simulink model "main"  (R2021a)
settings: Solver=ode113  StartTime=0.0  StopTime=300  RelTol=1e-13  AbsTol=1e-14
values from neighbouring files (symbols this model uses):
  Const = createSimulinkBus(Const_1)    [initializeData.m]
  Earth = createSimulinkBus(Earth_1)    [initializeData.m]
  Sensors = createSimulinkBus(Sensors_1)    [initializeData.m]
  Spacecraft = createSimulinkBus(Spacecraft_1)    [initializeData.m]
  totalTorque = [0 0 0 0.000704944678681 0.000834848489248 0.000628617928475 0.000704944678681 -0.000834848489248 -0.000628617928475 0.00140988935736 0 0 ... (48 elements, 3x16)]    [totalTorque.mat]
undefined symbols (not defined in the file or in its folder): initCond, torqueLookUpTable
libraries: simulink x22, SADlibrary x22, aerolibutil x20, vrlib x14, dspsrcs4 x12, sharedtransform x5, commfilt2 x3, dspfdesign x3, simulink_extras x2, sharedTrackingLibrary x2, dspmathops x1, sharedutil x1
(part 2 of 2)

== system main/Star sensor/Vector 2 angles ==
  In1 : Inport
  Atan1 : Trigonometry  Operator=atan2
  Atan2 : Trigonometry  Operator=atan2
  Demux : Demux  Outputs=3
  Mux : Mux  Inputs=2
  Random Source : dspsrcs4/Random Source  SrcType=Gaussian  NormMethod=Ziggurat  CltLength=12  MinVal=0  MaxVal=1  MeanVal=0  VarVal=Sensors.starTrackerCovariance  RepMode=Not repeatable  rawSeed=1  IsInherit=off  SampMode=Discrete  SampTime=1/Sensors.starTrackerSamplingFreq  SampFrame=2  DataType=Double  OutComplex=Real  OutputFrames=off
  Sum : Sum  Inputs=|++
  Star 1 : Outport
  wires:
  In1/1 -> Demux/1
  Sum/1 -> Star 1/1
  Mux/1 -> Sum/1
  Atan1/1 -> Mux/2
  Random Source/1 -> Sum/2
  Demux/3 -> Atan2/2, Atan1/2
  Atan2/1 -> Mux/1
  Demux/2 -> Atan1/1
  Demux/1 -> Atan2/1

== system main/Star sensor/Vector 2 angles1 ==
  In1 : Inport
  Atan1 : Trigonometry  Operator=atan2
  Atan2 : Trigonometry  Operator=atan2
  Demux : Demux  Outputs=3
  Mux : Mux  Inputs=2
  Random Source : dspsrcs4/Random Source  SrcType=Gaussian  NormMethod=Ziggurat  CltLength=12  MinVal=0  MaxVal=1  MeanVal=0  VarVal=Sensors.starTrackerCovariance  RepMode=Not repeatable  rawSeed=1  IsInherit=off  SampMode=Discrete  SampTime=1/Sensors.starTrackerSamplingFreq  SampFrame=2  DataType=Double  OutComplex=Real  OutputFrames=off
  Sum : Sum  Inputs=|++
  Star 1 : Outport
  wires:
  In1/1 -> Demux/1
  Sum/1 -> Star 1/1
  Mux/1 -> Sum/1
  Atan1/1 -> Mux/2
  Random Source/1 -> Sum/2
  Demux/3 -> Atan2/2, Atan1/2
  Atan2/1 -> Mux/1
  Demux/2 -> Atan1/1
  Demux/1 -> Atan2/1

== system main/Star sensor/Vector 2 angles2 ==
  In1 : Inport
  Atan1 : Trigonometry  Operator=atan2
  Atan2 : Trigonometry  Operator=atan2
  Demux : Demux  Outputs=3
  Mux : Mux  Inputs=2
  Random Source : dspsrcs4/Random Source  SrcType=Gaussian  NormMethod=Ziggurat  CltLength=12  MinVal=0  MaxVal=1  MeanVal=0  VarVal=Sensors.starTrackerCovariance  RepMode=Not repeatable  rawSeed=1  IsInherit=off  SampMode=Discrete  SampTime=1/Sensors.starTrackerSamplingFreq  SampFrame=2  DataType=Double  OutComplex=Real  OutputFrames=off
  Sum : Sum  Inputs=|++
  Star 1 : Outport
  wires:
  In1/1 -> Demux/1
  Sum/1 -> Star 1/1
  Mux/1 -> Sum/1
  Atan1/1 -> Mux/2
  Random Source/1 -> Sum/2
  Demux/3 -> Atan2/2, Atan1/2
  Atan2/1 -> Mux/1
  Demux/2 -> Atan1/1
  Demux/1 -> Atan2/1

== system main/Star sensor/Vector 2 angles3 ==
  In1 : Inport
  Atan1 : Trigonometry  Operator=atan2
  Atan2 : Trigonometry  Operator=atan2
  Demux : Demux  Outputs=3
  Mux : Mux  Inputs=2
  Random Source : dspsrcs4/Random Source  SrcType=Gaussian  NormMethod=Ziggurat  CltLength=12  MinVal=0  MaxVal=1  MeanVal=0  VarVal=Sensors.starTrackerCovariance  RepMode=Not repeatable  rawSeed=1  IsInherit=off  SampMode=Discrete  SampTime=1/Sensors.starTrackerSamplingFreq  SampFrame=2  DataType=Double  OutComplex=Real  OutputFrames=off
  Sum : Sum  Inputs=|++
  Star 1 : Outport
  wires:
  In1/1 -> Demux/1
  Sum/1 -> Star 1/1
  Mux/1 -> Sum/1
  Atan1/1 -> Mux/2
  Random Source/1 -> Sum/2
  Demux/3 -> Atan2/2, Atan1/2
  Atan2/1 -> Mux/1
  Demux/2 -> Atan1/1
  Demux/1 -> Atan2/1

== system main/State estimator/State 2 attitude and bias ==
  xHat : Inport
  Demux1 : Demux  Outputs=7
  Mux2 : Mux
  Mux3 : Mux  Inputs=3
  Body frame attitude [ECI] : Outport
  Gyro bias [body frame] : Outport  Port=2
  wires:
  Mux2/1 -> Body frame attitude [ECI]/1
  Demux1/2 -> Mux2/2
  Mux3/1 -> Gyro bias [body frame]/1
  Demux1/7 -> Mux3/3
  Demux1/1 -> Mux2/1
  Demux1/3 -> Mux2/3
  Demux1/5 -> Mux3/1
  xHat/1 -> Demux1/1
  Demux1/6 -> Mux3/2
  Demux1/4 -> Mux2/4

== system main/State estimator/State 2 attitude and bias1 ==
  xHat : Inport
  Demux1 : Demux  Outputs=7
  Mux2 : Mux
  Mux3 : Mux  Inputs=3
  Body frame attitude [ECI] : Outport
  Gyro bias [body frame] : Outport  Port=2
  wires:
  Mux2/1 -> Body frame attitude [ECI]/1
  Demux1/2 -> Mux2/2
  Mux3/1 -> Gyro bias [body frame]/1
  Demux1/7 -> Mux3/3
  Demux1/1 -> Mux2/1
  Demux1/3 -> Mux2/3
  Demux1/5 -> Mux3/1
  xHat/1 -> Demux1/1
  Demux1/6 -> Mux3/2
  Demux1/4 -> Mux2/4

== system main/Subsystem/Vec norm ==
  Vector : Inport
  Sqrt1 : Sqrt  SaturateOnIntegerOverflow=on
  Square : Math  Operator=square  SaturateOnIntegerOverflow=on
  Sum of Elements : Sum  Inputs=+
  Length : Outport
  wires:
  Sqrt1/1 -> Length/1
  Sum of Elements/1 -> Sqrt1/1
  Vector/1 -> Square/1
  Square/1 -> Sum of Elements/1

== system main/Subsystem/Vec norm1 ==
  Vector : Inport
  Sqrt1 : Sqrt  SaturateOnIntegerOverflow=on
  Square : Math  Operator=square  SaturateOnIntegerOverflow=on
  Sum of Elements : Sum  Inputs=+
  Length : Outport
  wires:
  Sqrt1/1 -> Length/1
  Sum of Elements/1 -> Sqrt1/1
  Vector/1 -> Square/1
  Square/1 -> Sum of Elements/1

== system main/Subsystem/Vec norm2 ==
  Vector : Inport
  Sqrt1 : Sqrt  SaturateOnIntegerOverflow=on
  Square : Math  Operator=square  SaturateOnIntegerOverflow=on
  Sum of Elements : Sum  Inputs=+
  Length : Outport
  wires:
  Sqrt1/1 -> Length/1
  Sum of Elements/1 -> Sqrt1/1
  Vector/1 -> Square/1
  Square/1 -> Sum of Elements/1

== system main/Subsystem1/Sun sensor reading1 ==
  True Sun position [body reference frame][km] : Inport  OutDataTypeStr=double  Unit=km
  Atan1 : Trigonometry  Operator=atan2
  Atan2 : Trigonometry  Operator=atan2
  Constant : Constant  Value=0*.5*pi/180*randn(2,1)
  Demux1 : Demux  Outputs=3
  Mux : Mux  Inputs=2
  Normalize Vector : vrlib/Utilities/Normalize Vector  maxzero=0
  Quaternion Rotation : aerolibutil/Quaternion Rotation
  Random Source1 : dspsrcs4/Random Source  SrcType=Gaussian  NormMethod=Ziggurat  CltLength=12  MinVal=0  MaxVal=1  MeanVal=0  VarVal=(.1*pi/180)^2  RepMode=Not repeatable  rawSeed=1  IsInherit=off  SampMode=Discrete  SampTime=Sensors.sunSensorSamplingFreq  SampFrame=2  DataType=Double  OutComplex=Real  OutputFrames=off
  Saturation : Saturate  UpperLimit=60*pi/180  LowerLimit=-60*pi/180
  Sensor orientation : Constant  Value=[1 0 0 0]
  Sum : Sum  Inputs=|++
  Sum1 : Sum  Inputs=++|
  Zero-Order Hold : ZeroOrderHold  SampleTime=Sensors.sunSensorSamplingFreq
  Sun angles position [sensor axis] : Outport  OutDataTypeStr=double  Unit=1
  wires:
  True Sun position [body reference frame][km]/1 -> Zero-Order Hold/1
  Sensor orientation/1 -> Quaternion Rotation/1
  Zero-Order Hold/1 -> Normalize Vector/1
  Normalize Vector/1 -> Quaternion Rotation/2
  Quaternion Rotation/1 -> Demux1/1
  Demux1/1 -> Atan2/1
  Demux1/3 -> Atan1/2, Atan2/2
  Demux1/2 -> Atan1/1
  Atan2/1 -> Mux/1
  Atan1/1 -> Mux/2
  Constant/1 -> Sum1/1
  Mux/1 -> Sum1/2
  Saturation/1 -> Sun angles position [sensor axis]/1
  Random Source1/1 -> Sum/2
  Sum/1 -> Saturation/1
  Sum1/1 -> Sum/1

== system main/Subsystem1/Sun sensor reading2 ==
  True Sun position [body reference frame][km] : Inport  OutDataTypeStr=double  Unit=km
  Atan1 : Trigonometry  Operator=atan2
  Atan2 : Trigonometry  Operator=atan2
  Constant : Constant  Value=0*.5*pi/180*randn(2,1)
  Demux1 : Demux  Outputs=3
  Mux : Mux  Inputs=2
  Normalize Vector : vrlib/Utilities/Normalize Vector  maxzero=0
  Quaternion Rotation : aerolibutil/Quaternion Rotation
  Random Source1 : dspsrcs4/Random Source  SrcType=Gaussian  NormMethod=Ziggurat  CltLength=12  MinVal=0  MaxVal=1  MeanVal=0  VarVal=(.1*pi/180)^2  RepMode=Not repeatable  rawSeed=1  IsInherit=off  SampMode=Discrete  SampTime=Sensors.sunSensorSamplingFreq  SampFrame=2  DataType=Double  OutComplex=Real  OutputFrames=off
  Saturation : Saturate  UpperLimit=60*pi/180  LowerLimit=-60*pi/180
  Sensor orientation : Constant  Value=[cos(pi/4) sin(pi/4) 0 0]
  Sum : Sum  Inputs=|++
  Sum1 : Sum  Inputs=++|
  Zero-Order Hold : ZeroOrderHold  SampleTime=Sensors.sunSensorSamplingFreq
  Sun angles position [sensor axis] : Outport  OutDataTypeStr=double  Unit=1
  wires:
  True Sun position [body reference frame][km]/1 -> Zero-Order Hold/1
  Sensor orientation/1 -> Quaternion Rotation/1
  Zero-Order Hold/1 -> Normalize Vector/1
  Normalize Vector/1 -> Quaternion Rotation/2
  Quaternion Rotation/1 -> Demux1/1
  Demux1/1 -> Atan2/1
  Demux1/3 -> Atan1/2, Atan2/2
  Demux1/2 -> Atan1/1
  Atan2/1 -> Mux/1
  Atan1/1 -> Mux/2
  Constant/1 -> Sum1/1
  Mux/1 -> Sum1/2
  Saturation/1 -> Sun angles position [sensor axis]/1
  Random Source1/1 -> Sum/2
  Sum/1 -> Saturation/1
  Sum1/1 -> Sum/1

== system main/Subsystem1/Sun sensor reading3 ==
  True Sun position [body reference frame][km] : Inport  OutDataTypeStr=double  Unit=km
  Atan1 : Trigonometry  Operator=atan2
  Atan2 : Trigonometry  Operator=atan2
  Constant : Constant  Value=0*.5*pi/180*randn(2,1)
  Demux1 : Demux  Outputs=3
  Mux : Mux  Inputs=2
  Normalize Vector : vrlib/Utilities/Normalize Vector  maxzero=0
  Quaternion Rotation : aerolibutil/Quaternion Rotation
  Random Source1 : dspsrcs4/Random Source  SrcType=Gaussian  NormMethod=Ziggurat  CltLength=12  MinVal=0  MaxVal=1  MeanVal=0  VarVal=(.1*pi/180)^2  RepMode=Not repeatable  rawSeed=1  IsInherit=off  SampMode=Discrete  SampTime=Sensors.sunSensorSamplingFreq  SampFrame=2  DataType=Double  OutComplex=Real  OutputFrames=off
  Saturation : Saturate  UpperLimit=60*pi/180  LowerLimit=-60*pi/180
  Sensor orientation : Constant  Value=[cos(pi/2) sin(pi/2) 0 0]
  Sum : Sum  Inputs=|++
  Sum1 : Sum  Inputs=++|
  Zero-Order Hold : ZeroOrderHold  SampleTime=Sensors.sunSensorSamplingFreq
  Sun angles position [sensor axis] : Outport  OutDataTypeStr=double  Unit=1
  wires:
  True Sun position [body reference frame][km]/1 -> Zero-Order Hold/1
  Sensor orientation/1 -> Quaternion Rotation/1
  Zero-Order Hold/1 -> Normalize Vector/1
  Normalize Vector/1 -> Quaternion Rotation/2
  Quaternion Rotation/1 -> Demux1/1
  Demux1/1 -> Atan2/1
  Demux1/3 -> Atan1/2, Atan2/2
  Demux1/2 -> Atan1/1
  Atan2/1 -> Mux/1
  Atan1/1 -> Mux/2
  Constant/1 -> Sum1/1
  Mux/1 -> Sum1/2
  Saturation/1 -> Sun angles position [sensor axis]/1
  Random Source1/1 -> Sum/2
  Sum/1 -> Saturation/1
  Sum1/1 -> Sum/1

== system main/Subsystem1/Sun sensor reading4 ==
  True Sun position [body reference frame][km] : Inport  OutDataTypeStr=double  Unit=km
  Atan1 : Trigonometry  Operator=atan2
  Atan2 : Trigonometry  Operator=atan2
  Constant : Constant  Value=0*.5*pi/180*randn(2,1)
  Demux1 : Demux  Outputs=3
  Mux : Mux  Inputs=2
  Normalize Vector : vrlib/Utilities/Normalize Vector  maxzero=0
  Quaternion Rotation : aerolibutil/Quaternion Rotation
  Random Source1 : dspsrcs4/Random Source  SrcType=Gaussian  NormMethod=Ziggurat  CltLength=12  MinVal=0  MaxVal=1  MeanVal=0  VarVal=(.1*pi/180)^2  RepMode=Not repeatable  rawSeed=1  IsInherit=off  SampMode=Discrete  SampTime=Sensors.sunSensorSamplingFreq  SampFrame=2  DataType=Double  OutComplex=Real  OutputFrames=off
  Saturation : Saturate  UpperLimit=60*pi/180  LowerLimit=-60*pi/180
  Sensor orientation : Constant  Value=[cos(pi/4) -sin(pi/4) 0 0]
  Sum : Sum  Inputs=|++
  Sum1 : Sum  Inputs=++|
  Zero-Order Hold : ZeroOrderHold  SampleTime=Sensors.sunSensorSamplingFreq
  Sun angles position [sensor axis] : Outport  OutDataTypeStr=double  Unit=1
  wires:
  True Sun position [body reference frame][km]/1 -> Zero-Order Hold/1
  Sensor orientation/1 -> Quaternion Rotation/1
  Zero-Order Hold/1 -> Normalize Vector/1
  Normalize Vector/1 -> Quaternion Rotation/2
  Quaternion Rotation/1 -> Demux1/1
  Demux1/1 -> Atan2/1
  Demux1/3 -> Atan1/2, Atan2/2
  Demux1/2 -> Atan1/1
  Atan2/1 -> Mux/1
  Atan1/1 -> Mux/2
  Constant/1 -> Sum1/1
  Mux/1 -> Sum1/2
  Saturation/1 -> Sun angles position [sensor axis]/1
  Random Source1/1 -> Sum/2
  Sum/1 -> Saturation/1
  Sum1/1 -> Sum/1

== system main/Subsystem1/Sun sensor reading5 ==
  True Sun position [body reference frame][km] : Inport  OutDataTypeStr=double  Unit=km
  Atan1 : Trigonometry  Operator=atan2
  Atan2 : Trigonometry  Operator=atan2
  Constant : Constant  Value=0*.5*pi/180*randn(2,1)
  Demux1 : Demux  Outputs=3
  Mux : Mux  Inputs=2
  Normalize Vector : vrlib/Utilities/Normalize Vector  maxzero=0
  Quaternion Rotation : aerolibutil/Quaternion Rotation
  Random Source1 : dspsrcs4/Random Source  SrcType=Gaussian  NormMethod=Ziggurat  CltLength=12  MinVal=0  MaxVal=1  MeanVal=0  VarVal=(.1*pi/180)^2  RepMode=Not repeatable  rawSeed=1  IsInherit=off  SampMode=Discrete  SampTime=Sensors.sunSensorSamplingFreq  SampFrame=2  DataType=Double  OutComplex=Real  OutputFrames=off
  Saturation : Saturate  UpperLimit=60*pi/180  LowerLimit=-60*pi/180
  Sensor orientation : Constant  Value=[cos(pi/4) 0 sin(pi/4) 0]
  Sum : Sum  Inputs=|++
  Sum1 : Sum  Inputs=++|
  Zero-Order Hold : ZeroOrderHold  SampleTime=Sensors.sunSensorSamplingFreq
  Sun angles position [sensor axis] : Outport  OutDataTypeStr=double  Unit=1
  wires:
  True Sun position [body reference frame][km]/1 -> Zero-Order Hold/1
  Sensor orientation/1 -> Quaternion Rotation/1
  Zero-Order Hold/1 -> Normalize Vector/1
  Normalize Vector/1 -> Quaternion Rotation/2
  Quaternion Rotation/1 -> Demux1/1
  Demux1/1 -> Atan2/1
  Demux1/3 -> Atan1/2, Atan2/2
  Demux1/2 -> Atan1/1
  Atan2/1 -> Mux/1
  Atan1/1 -> Mux/2
  Constant/1 -> Sum1/1
  Mux/1 -> Sum1/2
  Saturation/1 -> Sun angles position [sensor axis]/1
  Random Source1/1 -> Sum/2
  Sum/1 -> Saturation/1
  Sum1/1 -> Sum/1

== system main/Subsystem1/Sun sensor reading6 ==
  True Sun position [body reference frame][km] : Inport  OutDataTypeStr=double  Unit=km
  Atan1 : Trigonometry  Operator=atan2
  Atan2 : Trigonometry  Operator=atan2
  Constant : Constant  Value=0*.5*pi/180*randn(2,1)
  Demux1 : Demux  Outputs=3
  Mux : Mux  Inputs=2
  Normalize Vector : vrlib/Utilities/Normalize Vector  maxzero=0
  Quaternion Rotation : aerolibutil/Quaternion Rotation
  Random Source1 : dspsrcs4/Random Source  SrcType=Gaussian  NormMethod=Ziggurat  CltLength=12  MinVal=0  MaxVal=1  MeanVal=0  VarVal=(.1*pi/180)^2  RepMode=Not repeatable  rawSeed=1  IsInherit=off  SampMode=Discrete  SampTime=Sensors.sunSensorSamplingFreq  SampFrame=2  DataType=Double  OutComplex=Real  OutputFrames=off
  Saturation : Saturate  UpperLimit=60*pi/180  LowerLimit=-60*pi/180
  Sensor orientation : Constant  Value=[cos(pi/4) 0 -sin(pi/4) 0]
  Sum : Sum  Inputs=|++
  Sum1 : Sum  Inputs=++|
  Zero-Order Hold : ZeroOrderHold  SampleTime=Sensors.sunSensorSamplingFreq
  Sun angles position [sensor axis] : Outport  OutDataTypeStr=double  Unit=1
  wires:
  True Sun position [body reference frame][km]/1 -> Zero-Order Hold/1
  Sensor orientation/1 -> Quaternion Rotation/1
  Zero-Order Hold/1 -> Normalize Vector/1
  Normalize Vector/1 -> Quaternion Rotation/2
  Quaternion Rotation/1 -> Demux1/1
  Demux1/1 -> Atan2/1
  Demux1/3 -> Atan1/2, Atan2/2
  Demux1/2 -> Atan1/1
  Atan2/1 -> Mux/1
  Atan1/1 -> Mux/2
  Constant/1 -> Sum1/1
  Mux/1 -> Sum1/2
  Saturation/1 -> Sun angles position [sensor axis]/1
  Random Source1/1 -> Sum/2
  Sum/1 -> Saturation/1
  Sum1/1 -> Sum/1

== system main/Real physics/Air drag/Air density ==
  note: Because the density is a continuous function it doesn't matter if with an Height equal to a breakpoint value (e.g. =700km) we consider a base height of 700km or a base height of 600km
  Height : Inport
  1-D Lookup Base height : Lookup_n-D  NumberOfTableDimensions=1  BreakpointsForDimension1=Earth.atm_referenceHeight  IndexSearchMethod=Evenly spaced points  BeginIndexSearchUsingPreviousIndexResult=on  Table=Earth.atm_referenceHeight  InterpMethod=Flat  ExtrapMethod=Clip  UseLastTableValue=on  InternalRulePriority=Speed  RndMeth=Simplest  InputSameDT=on
  1-D Lookup Nominal density : Lookup_n-D  NumberOfTableDimensions=1  BreakpointsForDimension1=Earth.atm_referenceHeight  IndexSearchMethod=Evenly spaced points  BeginIndexSearchUsingPreviousIndexResult=on  Table=Earth.atm_nominalDensity  InterpMethod=Flat  InternalRulePriority=Speed  RndMeth=Simplest  InputSameDT=on
  1-D Lookup Scale height : Lookup_n-D  NumberOfTableDimensions=1  BreakpointsForDimension1=Earth.atm_referenceHeight  IndexSearchMethod=Evenly spaced points  BeginIndexSearchUsingPreviousIndexResult=on  Table=Earth.atm_scaleHeight  InterpMethod=Flat  InternalRulePriority=Speed  RndMeth=Simplest  InputSameDT=on
  Divide : Product  Inputs=*/
  Exp : Math  SaturateOnIntegerOverflow=on
  Product : Product
  Sum : Sum  Inputs=-+|
  Air density : Outport
  wires:
  Height/1 -> 1-D Lookup Nominal density/1, 1-D Lookup Scale height/1, 1-D Lookup Base height/1, Sum/1
  1-D Lookup Nominal density/1 -> Product/2
  1-D Lookup Base height/1 -> Sum/2
  Sum/1 -> Divide/1
  1-D Lookup Scale height/1 -> Divide/2
  Divide/1 -> Exp/1
  Product/1 -> Air density/1
  Exp/1 -> Product/1

== system main/Real physics/Magnetic effect (torque only)/Cartesian to polar ==
  Unitary vector [cartesian coord] : Inport
  Atan1 : Trigonometry  Operator=atan2
  Atan2 : Trigonometry  Operator=atan2
  Demux : Demux  Outputs=3
  Sqrt : Sqrt  SaturateOnIntegerOverflow=on
  Square : Math  Operator=square  SaturateOnIntegerOverflow=on
  Square1 : Math  Operator=square  SaturateOnIntegerOverflow=on
  Sum : Sum
  Colatitude - θ : Outport
  Longitude - φ : Outport  Port=2
  wires:
  Demux/2 -> Square1/1, Atan2/1
  Square/1 -> Sum/1
  Square1/1 -> Sum/2
  Atan1/1 -> Colatitude - θ/1
  Sum/1 -> Sqrt/1
  Unitary vector [cartesian coord]/1 -> Demux/1
  Demux/1 -> Square/1, Atan2/2
  Demux/3 -> Atan1/2
  Atan2/1 -> Longitude - φ/1
  Sqrt/1 -> Atan1/1

== system main/Real physics/Rotational dynamic/Euler equations (rigid body)  ==
  note: $\dot\mathbf{\Gamma} = \left[ (-I_z+I_y) \omega_y \omega_z \quad (-I_x+I_z) \omega_z \omega_x \quad \right (-I_y+I_x) \omega_x \omega_y]^T$
      |
      | Please note that
      | $\left[b \quad c \quad a \right] = \text{Cycle_3_vector}\left([a \quad b \quad c]\right)$
  omega [body reference frame] : Inport
  Inertia [body reference frame] : Inport  Port=2  Unit=kg*m^2
  External torque [body reference frame] : Inport  Port=3  Unit=N*m
  Cycle vector{,1..3} (4 alike) : SADlibrary/Cycle vector  SystemSampleTime=-1  VariantActivationTime=update diagram  Latency=0  AutoFrameSizeCalculation=off
  Divide : Product  Inputs=*/
  Product : Product  Inputs=3
  Sum : Sum  Inputs=++|
  Sum1 : Sum  Inputs=|-+
  omega dot [body reference frame] : Outport
  wires:
  Inertia [body reference frame]/1 -> Cycle vector2/1, Divide/2
  External torque [body reference frame]/1 -> Sum/1
  Sum/1 -> Divide/1
  Divide/1 -> omega dot [body reference frame]/1
  omega [body reference frame]/1 -> Cycle vector/1
  Cycle vector2/1 -> Cycle vector3/1, Sum1/1
  Cycle vector3/1 -> Sum1/2
  Cycle vector/1 -> Cycle vector1/1, Product/2
  Cycle vector1/1 -> Product/1
  Sum1/1 -> Product/3
  Product/1 -> Sum/2

== system main/Real physics/Rotational dynamic/Kinematics with quaternions ==
  q : Inport  Unit=1
  omega [body frame] : Inport  Port=2  Unit=rad/s
  Gain1 : Gain  Gain=1/2
  MATLAB Function1 : MATLAB Function  TreatAsAtomicUnit=on
  Matrix Multiply : Product  Multiplication=Matrix(*)
  q dot : Outport
  wires:
  omega [body frame]/1 -> MATLAB Function1/1(omega)
  Gain1/1 -> Matrix Multiply/1
  Matrix Multiply/1 -> q dot/1
  MATLAB Function1/1(Omega) -> Gain1/1
  q/1 -> Matrix Multiply/2

== system main/Real physics/Solar radiation pressure (torque only)/Solar radiation pressure ==
  Distance from the sun : Inport  Unit=km
  1AU [km] : Constant  Value=Const.AU_1
  Divide : Product  Inputs=*/
  Divide1 : Product  Inputs=*/
  Fe [W/m^2] : Constant  Value=Const.Fe
  Product : Product
  Square : Math  Operator=square  SaturateOnIntegerOverflow=on
  c [m/s] : Constant  Value=Const.c
  SRP : Outport  Unit=Pa
  wires:
  1AU [km]/1 -> Divide/1
  Distance from the sun/1 -> Divide/2
  Divide/1 -> Square/1
  Fe [W/m^2]/1 -> Divide1/1
  c [m/s]/1 -> Divide1/2
  Square/1 -> Product/1
  Divide1/1 -> Product/2
  Product/1 -> SRP/1

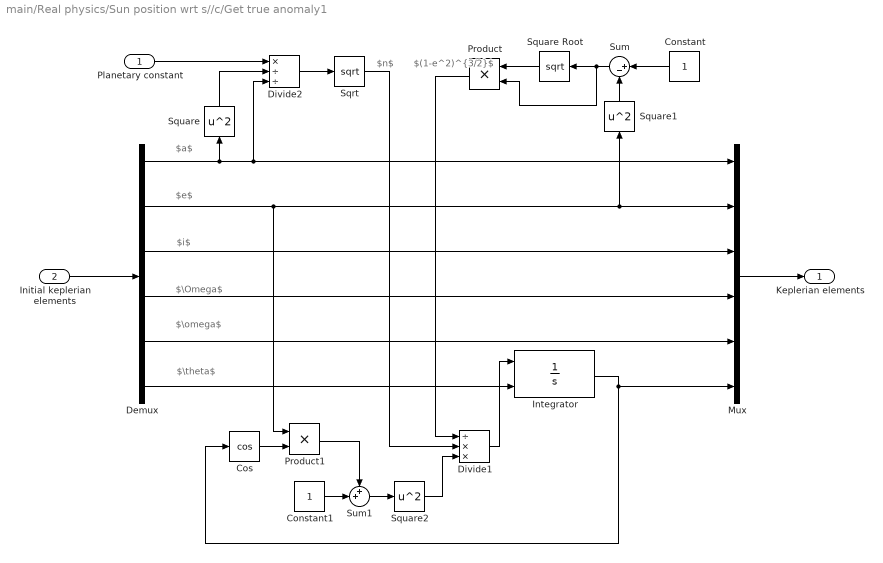
== system main/Real physics/Sun position wrt s//c/Get true anomaly1 ==
  note: $(1-e^2)^{3/2}$
  note: $n$
  note: $\theta$
  note: $\omega$
  note: $\Omega$
  note: $i$
  note: $e$
  note: $a$
  Planetary constant : Inport
  Initial keplerian elements : Inport  Port=2
  Constant : Constant
  Constant1 : Constant
  Cos : Trigonometry  Operator=cos
  Demux : Demux  Outputs=6
  Divide1 : Product  Inputs=/**
  Divide2 : Product  Inputs=*//
  Integrator : Integrator  InitialConditionSource=external
  Mux : Mux  Inputs=6
  Product : Product
  Product1 : Product
  Sqrt : Sqrt  SaturateOnIntegerOverflow=on
  Square : Math  Operator=square  SaturateOnIntegerOverflow=on
  Square Root : Sqrt  SaturateOnIntegerOverflow=on
  Square1 : Math  Operator=square  SaturateOnIntegerOverflow=on
  Square2 : Math  Operator=square  SaturateOnIntegerOverflow=on
  Sum : Sum  Inputs=|+-
  Sum1 : Sum  Inputs=++|
  Keplerian elements : Outport
  wires:
  Initial keplerian elements/1 -> Demux/1
  Mux/1 -> Keplerian elements/1
  Demux/1 -> Square/1, Divide2/3, Mux/1
  Demux/2 -> Mux/2, Square1/1, Product1/1
  Demux/3 -> Mux/3
  Demux/4 -> Mux/4
  Demux/5 -> Mux/5
  Demux/6 -> Integrator/2
  Planetary constant/1 -> Divide2/1
  Square/1 -> Divide2/2
  Divide2/1 -> Sqrt/1
  Sqrt/1 -> Divide1/2
  Constant/1 -> Sum/1
  Square1/1 -> Sum/2
  Sum/1 -> Square Root/1, Product/2
  Square Root/1 -> Product/1
  Product/1 -> Divide1/1
  Cos/1 -> Product1/2
  Square2/1 -> Divide1/3
  Divide1/1 -> Integrator/1
  Constant1/1 -> Sum1/2
  Product1/1 -> Sum1/1
  Sum1/1 -> Square2/1
  Integrator/1 -> Mux/6, Cos/1

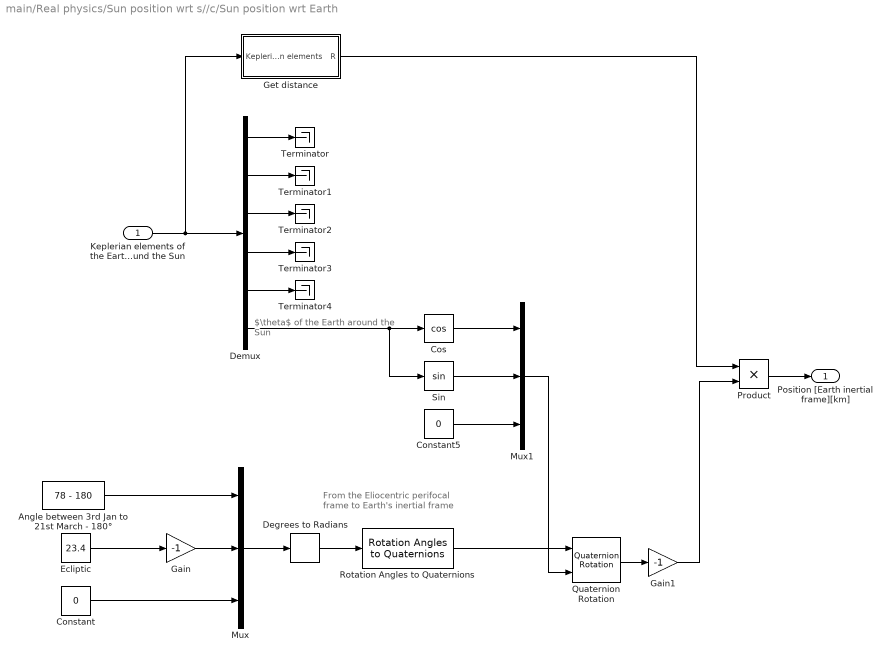
== system main/Real physics/Sun position wrt s//c/Sun position wrt Earth ==
  note: $\theta$ of the Earth around the Sun
  note: From the Eliocentric perifocal frame to Earth's inertial frame
  Keplerian elements of the Earth around the Sun : Inport
  Angle between 3rd Jan to 21st March - 180° : Constant  Value=78 - 180
  Constant : Constant  Value=0
  Constant5 : Constant  Value=0
  Cos : Trigonometry  Operator=cos
  Degrees to Radians : simulink_extras/Transformations/Degrees to Radians
  Demux : Demux  Outputs=6
  Ecliptic : Constant  Value=23.4
  Gain : Gain  Gain=-1
  Gain1 : Gain  Gain=-1
  Get distance : Subsystem
  Mux : Mux  Inputs=3
  Mux1 : Mux  Inputs=3
  Product : Product
  Quaternion Rotation : aerolibutil/Quaternion Rotation
  Rotation Angles to Quaternions : sharedtransform/Rotation Angles to Quaternions  rotationOrder=ZXY  aMode=aMode
      settings: SourceProductBaseCode=AE,PW,DR,MT,UV,VE
  Sin : Trigonometry
  Terminator{,1..4} (5 alike) : Terminator
  Position [Earth inertial frame][km] : Outport  Unit=km
  wires:
  Angle between 3rd Jan to 21st March - 180°/1 -> Mux/1
  Ecliptic/1 -> Gain/1
  Degrees to Radians/1 -> Rotation Angles to Quaternions/1
  Gain/1 -> Mux/2
  Constant/1 -> Mux/3
  Mux/1 -> Degrees to Radians/1
  Mux1/1 -> Quaternion Rotation/2
  Rotation Angles to Quaternions/1 -> Quaternion Rotation/1
  Quaternion Rotation/1 -> Gain1/1
  Gain1/1 -> Product/2
  Keplerian elements of the Earth around the Sun/1 -> Get distance/1(Keplerian elements), Demux/1
  Sin/1 -> Mux1/2
  Constant5/1 -> Mux1/3
  Cos/1 -> Mux1/1
  Demux/6 -> Sin/1, Cos/1
  Get distance/1(R) -> Product/1
  Demux/1 -> Terminator/1
  Demux/2 -> Terminator1/1
  Demux/3 -> Terminator2/1
  Demux/5 -> Terminator4/1
  Demux/4 -> Terminator3/1
  Product/1 -> Position [Earth inertial frame][km]/1

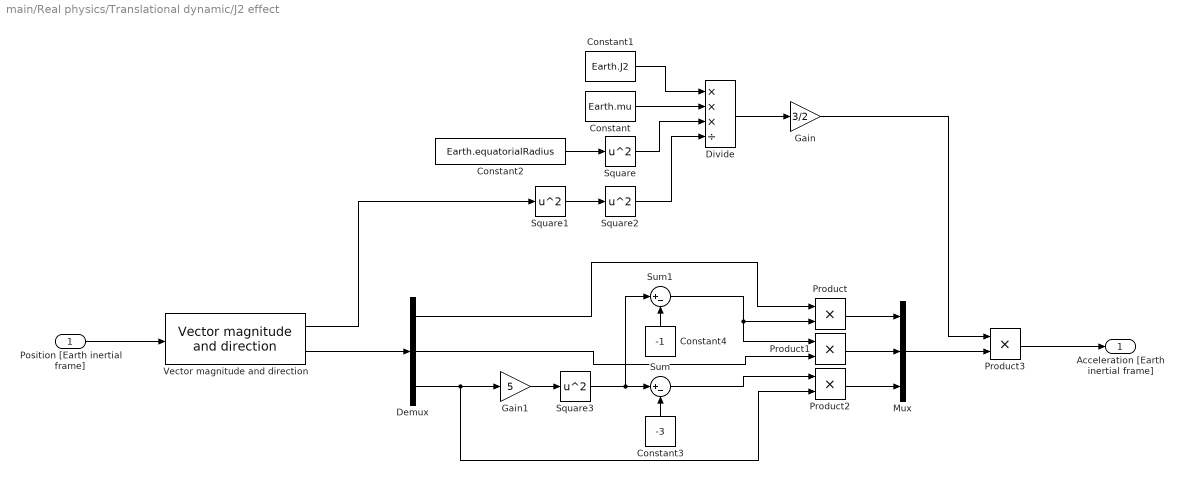
== system main/Real physics/Translational dynamic/J2 effect ==
  Position [Earth inertial frame] : Inport
  Constant : Constant  Value=Earth.mu
  Constant1 : Constant  Value=Earth.J2
  Constant2 : Constant  Value=Earth.equatorialRadius
  Constant3 : Constant  Value=-3
  Constant4 : Constant  Value=-1
  Demux : Demux  Outputs=3
  Divide : Product  Inputs=***/
  Gain : Gain  Gain=3/2
  Gain1 : Gain  Gain=5
  Mux : Mux  Inputs=3
  Product{,1..3} (4 alike) : Product
  Square{,1..3} (4 alike) : Math  Operator=square  SaturateOnIntegerOverflow=on
  Sum : Sum  Inputs=|+-
  Sum1 : Sum  Inputs=|+-
  Vector magnitude and direction : SADlibrary/Vector magnitude and direction  SystemSampleTime=-1  VariantActivationTime=update diagram  Latency=0  AutoFrameSizeCalculation=off
  Acceleration [Earth inertial frame] : Outport
  wires:
  Constant2/1 -> Square/1
  Constant1/1 -> Divide/1
  Constant/1 -> Divide/2
  Square/1 -> Divide/3
  Divide/1 -> Gain/1
  Square1/1 -> Square2/1
  Square2/1 -> Divide/4
  Vector magnitude and direction/1 -> Square1/1
  Position [Earth inertial frame]/1 -> Vector magnitude and direction/1
  Vector magnitude and direction/2 -> Demux/1
  Demux/3 -> Product2/2, Gain1/1
  Gain1/1 -> Square3/1
  Square3/1 -> Sum1/1, Sum/1
  Constant3/1 -> Sum/2
  Constant4/1 -> Sum1/2
  Product/1 -> Mux/1
  Product1/1 -> Mux/2
  Product2/1 -> Mux/3
  Sum1/1 -> Product1/1, Product/2
  Demux/1 -> Product/1
  Demux/2 -> Product1/2
  Sum/1 -> Product2/1
  Mux/1 -> Product3/2
  Product3/1 -> Acceleration [Earth inertial frame]/1
  Gain/1 -> Product3/1

== system main/Real physics/Translational dynamic/Main contribution ==
  Position [Earth inertial frame] : Inport
  Constant : Constant  Value=Earth.mu
  Divide : Product  Inputs=*/
  Gain : Gain  Gain=-1
  Product : Product
  Square : Math  Operator=square  SaturateOnIntegerOverflow=on
  Vector magnitude and direction : SADlibrary/Vector magnitude and direction  SystemSampleTime=-1  VariantActivationTime=update diagram  Latency=0  AutoFrameSizeCalculation=off
  Acceleration [Earth inertial frame] : Outport
  wires:
  Square/1 -> Divide/2
  Product/1 -> Acceleration [Earth inertial frame]/1
  Position [Earth inertial frame]/1 -> Vector magnitude and direction/1
  Divide/1 -> Gain/1
  Constant/1 -> Divide/1
  Vector magnitude and direction/1 -> Square/1
  Vector magnitude and direction/2 -> Product/2
  Gain/1 -> Product/1

== system main/Real physics/Sun position wrt s//c/Sun position wrt Earth/Get distance ==
  note: $\theta$
  note: $e$
  note: $a$
  Keplerian elements : Inport
  Constant : Constant
  Constant3 : Constant
  Cos : Trigonometry  Operator=cos
  Demux : Demux  Outputs=6
  Divide : Product  Inputs=*/
  Product : Product
  Product1 : Product
  Square : Math  Operator=square  SaturateOnIntegerOverflow=on
  Sum : Sum  Inputs=-|+
  Sum1 : Sum  Inputs=+|+
  Terminator : Terminator
  Terminator1 : Terminator
  Terminator2 : Terminator
  R : Outport
  wires:
  Keplerian elements/1 -> Demux/1
  Demux/1 -> Product/1
  Square/1 -> Sum/1
  Sum/1 -> Product/2
  Constant3/1 -> Sum/2
  Product/1 -> Divide/1
  Demux/2 -> Square/1, Product1/1
  Demux/6 -> Cos/1
  Cos/1 -> Product1/2
  Constant/1 -> Sum1/1
  Product1/1 -> Sum1/2
  Sum1/1 -> Divide/2
  Divide/1 -> R/1
  Demux/3 -> Terminator/1
  Demux/5 -> Terminator2/1
  Demux/4 -> Terminator1/1

== matlab function main/Ideal control law/MATLAB Function1 ==
  data: q input; e output
function e = fcn(q)

e = sqrt(q(2)^2+q(3)^2+q(4)^2) * 180 / pi * 2;

== matlab function main/Comparison/MATLAB Function2 ==
  data: q input; e output
function e = fcn(q)
e = sqrt(q(2)^2+q(3)^2+q(4)^2) * 180 / pi * 2;

== matlab function main/Solve Whabba's problem/MATLAB Function1 ==
  settings: updateMethod=DISCRETE
  data: K input; q output; qGuess input; err output
function [q,err] = getQ(K,qGuess)

q = qGuess;
err = 1;

for i=1:10 % err > 1e-6
    qOld = q;
    q = K*q;
    q = q/norm(q);
    err = sum((q - qOld).^2);
end

== matlab function main/Solve Whabba's problem/MATLAB Function2 ==
  data: S input; B output; V input
function B = computeBmatrix(S,V)%s1,v1,s2,v2,s3,v3)

B = zeros(3);%size(S,1));
for i=1:size(S,2)
    B = B + S(:,i)*V(:,i)';
end

% B = s1*v1'+s2*v2'+s3*v3';

== matlab function main/Solve Whabba's problem/MATLAB Function3 ==
  data: B input; A output
function A = BtoA(B)
[U,~,V] = svd(B);
M = diag([1 1 det(U)*det(V)]);
A = U*M*V';
%A = B \ sqrtm(B'*B);

== matlab function main/MATLAB Function1 ==
  data: lookUpTable input; t output; controlImpulse input
function t = fcn(lookUpTable,controlImpulse)
lambda = 1;
% First element
% w2 = dot(lookUpTable(1,13:15),lookUpTable(1,13:15));
% lambda = dot(controlImpulse,lookUpTable(1,13:15));
% lambda = lambda ./ w2;

deltaOpt = sum( abs(controlImpulse' - lambda .* lookUpTable(1,13:15)) ,2);
    
t = lookUpTable(1,13:15)';

% Others elements
for i=2:size(lookUpTable,2)
%     w2 = dot(lookUpTable(i,13:15),lookUpTable(i,13:15));
%     lambda = dot(controlImpulse,lookUpTable(i,13:15));
%     lambda = lambda ./ w2;
    
    delta2 = sum( abs(controlImpulse' - lambda .* lookUpTable(i,13:15)) ,2);
    
    if delta2 < deltaOpt
        deltaOpt = delta2;
        t = lookUpTable(i,13:15)';
    end
end

== matlab function main/Ideal control law/MATLAB Function2 ==
  data: J input; u output; torque input; omegaBody input; omegaErr input; qErr input; VdotMin output
function [u,VdotMin] = minLyapunov(J,torque,omegaBody,omegaErr,qErr)
%k1 = 1.5 * 1;
k2 = 1; %2 * 180/pi;

Vdot = @(M) omegaErr'*(M + cross(J.*omegaBody,omegaBody-omegaErr) + 2*k2*qErr(1)*qErr(2:4));

iMin = 1;
VdotMin = Vdot(torque(:,1));
for i=2:size(torque,2)
    if Vdot(torque(:,i)) < VdotMin
       iMin = i;
       VdotMin = Vdot(torque(:,i));
    end
end

u = torque(:,iMin);

== matlab function main/Control allocator/MATLAB Function3 ==
  data: cgtTorque input size=[3 4]; dGammaId input size=3; xOpt output size=4
function xOpt = controlAllocator(cgtTorque,dGammaId)

% dGammaId_x = zeros(3);
% dGammaId_x(:,1) = cross(dGammaId,[1 0 0]');
% dGammaId_x(:,2) = cross(dGammaId,[0 1 0]');
% dGammaId_x(:,3) = cross(dGammaId,[0 0 1]');

%A = dGammaId_x * cgtTorque;
%u = null(A);

% U = u'*u;
nThrusters = 4;
opt = optimoptions('lsqlin','Algorithm','active-set');
xOpt = lsqlin(cgtTorque,dGammaId,[],[],[],[],zeros(nThrusters,1),1/5*ones(nThrusters,1),zeros(nThrusters,1),opt);
% xOpt = quadprog(U,[],-u,zeros(12,1),[],[],[],[],[],[]);
% 
% uReal = u * xOpt;
% 
% dt = norm(dGammaId) / norm(cgtTorque*uReal);
% uTimes = dt * uReal;

== matlab function main/Real physics/Solar radiation pressure (torque only)/MATLAB Function ==
  data: sunDir input; F output; SRP input; Spacecraft input; T output
function [F,T] = SRTorque(sunDir,SRP,Spacecraft)
    % Spacecraft data
%     S = {(.1)^2,(.1)^2,(.1)^2,(.1)^2,(.1)^2,(.1)^2, 4.5*(.1)^2,4.5*(.1)^2,4.5*(.1)^2,4.5*(.1)^2};
%     surfNormVec = {[1;0;0],[0;1;0],[0;0;1],[-1;0;0],[0;-1;0],[0;0;-1], [1;0;0],[-1;0;0],[1;0;0],[-1;0;0]};
%     surfPosVec = {.1*[1;0;0],.1*[0;1;0],.1*[0;0;1],.1*[-1;0;0],.1*[0;-1;0],.1*[0;0;-1], .23*[0;1;0],.23*[0;1;0],.23*[0;-1;0],.23*[0;-1;0]};
    rhos = [.5,.5,.5,.5,.5,.5, .8,.8,.8,.8];
    rhod = [.1,.1,.1,.1,.1,.1, .1,.1,.1,.1];
    S = Spacecraft.surfaces_area;
    surfNormVec = Spacecraft.surfaces_normalToSurface;
    surfPosVec = Spacecraft.surfaces_position;
    geometricCenter = Spacecraft.geometricCenter;
    
    F = [0;0;0];
    T = [0;0;0];
    
    for i=1:numel(S)
       sunDir_dot_surfNormVec = dot(sunDir,surfNormVec(:,i));
       S_i = S(i);
       rhos_i = rhos(i);
       rhod_i = rhod(i);
       surfNormVec_i = surfNormVec(:,i);
       surfPosVec_i = surfPosVec(:,i);
       if sunDir_dot_surfNormVec > 0
           F_i = -SRP*S_i*sunDir_dot_surfNormVec*(...
               ( 1-rhos_i )*sunDir + ...
               ( 2/3*rhod_i+2*rhos_i*sunDir_dot_surfNormVec )*surfNormVec_i ...
               );
           F = F + F_i;
           T = T + cross(surfPosVec_i+geometricCenter,F_i);
       end
    end
end

== matlab function main/Real physics/Rotational dynamic/Kinematics with quaternions/MATLAB Function1 ==
  data: omega input size=[3 1]; Omega output size=[4 4]
function Omega = getOmega(omega)
    % Considering the quaternion q = a + i x + j y + k z
    % While in class we used the following convention:
    %   q_vec = [x y z a]'
    % MATLAB use a different convention:
    %   q_vec = [a x y z]'
    % For this reason the following matrix is different from the one we seen
    
    Omega = [         0 -omega(1)  -omega(2) -omega(3) ;
                      0         0   omega(3) -omega(2) ;
                      0         0          0  omega(1) ;
                      0         0          0         0 ];
    Omega = Omega - Omega';
end

== matlab function main/Real physics/Air drag/MATLAB Function ==
  data: F output; rho input; relVel input; T output; Spacecraft input
function [F,T] = getAirTorqueAndForce(rho, relVel, Spacecraft)

F = zeros(3,1);
T = zeros(3,1);

relVelMag = norm(relVel);
relVelDir = relVel/relVelMag;

for i = 1:size(Spacecraft.surfaces_normalToSurface,2)
    N_i = Spacecraft.surfaces_normalToSurface(:,i);
    A_i = Spacecraft.surfaces_area(:,i);
    r_i = Spacecraft.surfaces_position(:,i);
    Cd_i = Spacecraft.surfaces_Cd(i);
    
    F_i = dot(relVelDir,N_i);
    if F_i > 0
       F_i = F_i * 1/2*rho*Cd_i*relVelMag^2*A_i;
    else
       F_i = 0;
    end
    
    F = F - F_i * relVelDir;
    T = T - cross(r_i + Spacecraft.geometricCenter, F_i * relVelDir);
end

== matlab function main/MATLAB Function ==
  data: t input; q output; omega output
function [q,omega] = fcn(t)

om = 1/60; % 1/7200;
q = [cos(om*t/2) 0 0 sin(om*t/2)]';
omega = [0 0 1]'*om;

== matlab function main/Subsystem1/MATLAB Function1 ==
  data: s output size=[2 1]; s1 input; s2 input; s3 input; s4 input; s5 input; s6 input; sensAtt output
function [s,sensAtt] =  getSunSensorReading(s1,s2,s3,s4,s5,s6)
[~,i] = min([sum(s1.^2) sum(s2.^2) sum(s3.^2) sum(s4.^2) sum(s5.^2) sum(s6.^2)]);
switch i
    case 1
        s = s1;
        sensAtt = [1 0 0 0];
    case 2
        s = s2;
        sensAtt = [cos(pi/4) sin(pi/4) 0 0];
    case 3
        s = s3;
        sensAtt = [cos(pi/2) sin(pi/2) 0 0];
    case 4
        s = s4;
        sensAtt = [cos(pi/4) -sin(pi/4) 0 0];
    case 5
        s = s5;
        sensAtt = [cos(pi/4) 0 sin(pi/4) 0];
    case 6
        s = s6;
        sensAtt = [cos(pi/4) 0 -sin(pi/4) 0];
    otherwise
        error("Errore");
end

== matlab function main/Solve Whabba's problem/MATLAB Function4 ==
  data: sensorScreen input; S output; V output; in2 input
function [S,V] = fromSensorScreenToBodyFrame(sensorScreen,in2)
nStar = numel(sensorScreen)/2;

S = zeros(3,nStar);
V = zeros(3,nStar);

% From star sensor frame to body frame
q = in2(1:4);
R = [     1-2*q(3)^2-2*q(4)^2  2*q(2)*q(3)+2*q(1)*q(4) -2*q(1)*q(3)+2*q(2)*q(4) ;...
      2*q(2)*q(3)-2*q(1)*q(4)      1-2*q(2)^2-2*q(4)^2  2*q(1)*q(2)+2*q(3)*q(4) ;...
      2*q(1)*q(3)+2*q(2)*q(4) -2*q(1)*q(2)+2*q(3)*q(4)      1-2*q(2)^2-2*q(3)^2 ];

% Star in ECI
j = 1;
for i=5:3:(3*nStar+5)
    V(:,j) = in2(i:i+2);
    j = j+1;
end

% Star in body frame
j = 1;
for i=1:2:(2*nStar)
    S(:,j) = [tan(sensorScreen(i)) tan(sensorScreen(i+1)) 1]';
    S(:,j) = S(:,j) / norm(S(:,j));
    S(:,j) = R*S(:,j);
    j = j+1;
end

== matlab function main/Comparison/MATLAB Function ==
  data: q input; e output
function e = fcn(q)
e = sqrt(q(2)^2+q(3)^2+q(4)^2) * 180 / pi * 2;

== matlab function main/Comparison/MATLAB Function1 ==
  data: q input; e output
function e = fcn(q)
e = sqrt(q(2)^2+q(3)^2+q(4)^2) * 180 / pi * 2;

== matlab function main/Solve Whabba's problem/MATLAB Function ==
  data: B input; K output
function K = fromBtoK(B)
S = B+B';
sigma = trace(B);
Z = [B(2,3)-B(3,2) B(3,1)-B(1,3) B(1,2)-B(2,1)]';

K = [sigma             Z';...
         Z S-sigma*eye(3)];

== matlab function main/Ideal control law/MATLAB Function ==
  data: J input; omegaBody input; omegaErr input; u output; qErr input
function u = lyapunovControl(J,omegaBody,omegaErr,qErr)
k1 = 0.5 * 1;
k2 = 0.5 * 1;

% 2.5e-3
u = -k1 * omegaErr -2*k2 * qErr(1)*qErr(2:4) + cross(omegaBody-omegaErr,J.*omegaBody);
